simulink model "model_nff"  (R2014a)
settings: Solver=ode45  StartTime=0.0  StopTime=1000  RelTol=1e-3
values from neighbouring files (symbols this model uses):
  L5_final = 3.5    [regler_siso.m]
  L5_initial = 3    [regler_siso.m]
  L5_step = 500    [regler_siso.m]
  L7_final = 12.5    [regler_siso.m]
  L7_initial = 12    [regler_siso.m]
  L7_step = 500    [regler_siso.m]
libraries: cstblocks x4
settings Model: Creator=Nino  LastModifiedBy=Nino

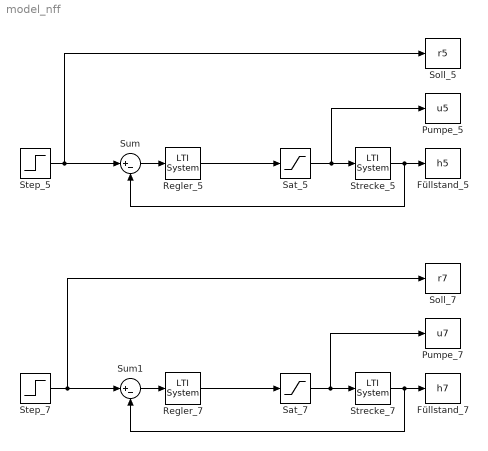
== system model_nff ==
  Füllstand_5 : ToWorkspace  VariableName=h5  SaveFormat=Structure With Time  SampleTime=-1
  Füllstand_7 : ToWorkspace  VariableName=h7  SaveFormat=Structure With Time  SampleTime=-1
  Pumpe_5 : ToWorkspace  VariableName=u5  SaveFormat=Structure With Time  SampleTime=-1
  Pumpe_7 : ToWorkspace  VariableName=u7  SaveFormat=Structure With Time  SampleTime=-1
  Regler_5 : cstblocks/LTI System  sys=C5  IC=[]
  Regler_7 : cstblocks/LTI System  sys=C7  IC=[]
  Sat_5 : Saturate  UpperLimit=10  LowerLimit=0
  Sat_7 : Saturate  UpperLimit=10  LowerLimit=0
  Soll_5 : ToWorkspace  VariableName=r5  SaveFormat=Structure With Time  SampleTime=-1
  Soll_7 : ToWorkspace  VariableName=r7  SaveFormat=Structure With Time  SampleTime=-1
  Step_5 : Step  Time=L5_step  Before=L5_initial  After=L5_final  SampleTime=0
  Step_7 : Step  Time=L7_step  Before=L7_initial  After=L7_final  SampleTime=0
  Strecke_5 : cstblocks/LTI System  sys=G5  IC=[]
  Strecke_7 : cstblocks/LTI System  sys=G7  IC=[]
  Sum : Sum  Inputs=|+-
  Sum1 : Sum  Inputs=|+-
  wires:
  Sat_5/1 -> Pumpe_5/1, Strecke_5/1
  Strecke_5/1 -> Füllstand_5/1, Sum/2
  Sum/1 -> Regler_5/1
  Step_5/1 -> Soll_5/1, Sum/1
  Sat_7/1 -> Pumpe_7/1, Strecke_7/1
  Strecke_7/1 -> Füllstand_7/1, Sum1/2
  Sum1/1 -> Regler_7/1
  Step_7/1 -> Soll_7/1, Sum1/1
  Regler_5/1 -> Sat_5/1
  Regler_7/1 -> Sat_7/1
